simulink model "buffer_tester"  (R2024b)
settings: Solver=ode1  StartTime=0.0  StopTime=100  FixedStep=0.05  RelTol=1e-3
libraries: buffer_lib x2, filter_lib x1, storage_lib x1
settings Model: Creator=marcv  LastModifiedBy=marcv
settings RTWCC: GPUComputeCapability=3.5

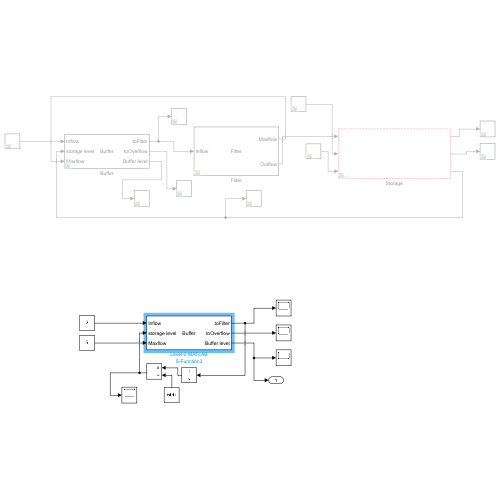
[thumbnail: Simulink's stored preview of the top-level diagram]
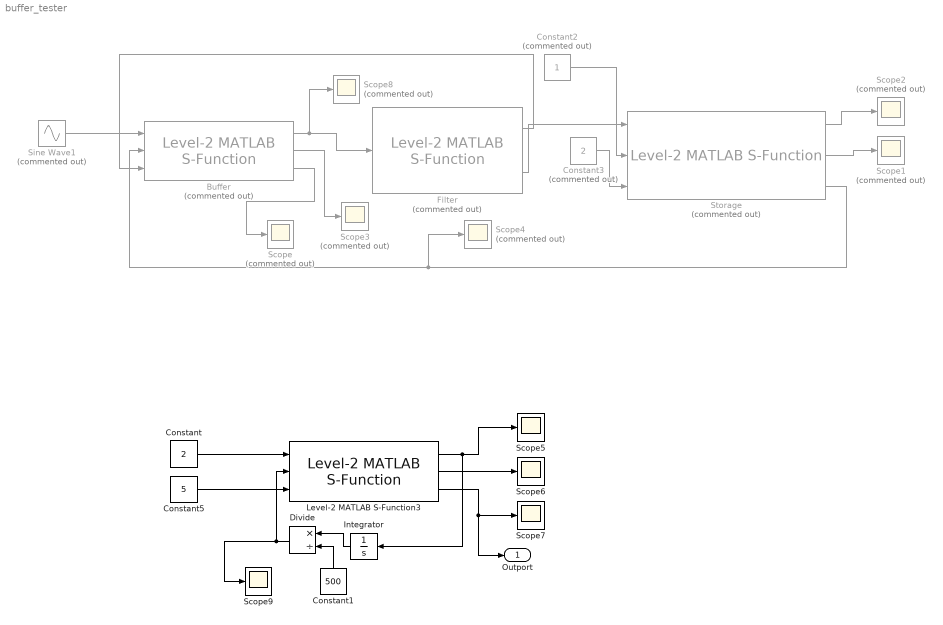
== system buffer_tester ==
  Buffer : buffer_lib/Level-2 MATLAB S-Function  Commented=on  Parameter1=100
  Constant : Constant  Value=2
  Constant1 : Constant  Value=500
  Constant2 : Constant  Commented=on
  Constant3 : Constant  Commented=on  Value=2
  Constant5 : Constant  Value=5
  Divide : Product  Inputs=*/
  Filter : filter_lib/Level-2 MATLAB S-Function  Commented=on  filteroption=Common filter  Parameter4=Cyclone-sand-UV [90 m3/h]  Parameter1=5  Parameter2=3
  Integrator : Integrator
  Level-2 MATLAB S-Function3 : buffer_lib/Level-2 MATLAB S-Function  Parameter1=1
  Scope{,1..4,8} (6 alike) : Scope  Commented=on
  Scope{5..7,9} (4 alike) : Scope
  Sine Wave1 : Sin  Commented=on  Amplitude=5  SampleTime=0
  Storage : storage_lib/Level-2 MATLAB S-Function  Commented=on  Parameter1=1000  Parameter2=0.20  Parameter3=No interconnection
  Outport : Outport
  wires:
  Sine Wave1/1 -> Buffer/1
  Buffer/2 -> Scope3/1
  Buffer/3 -> Scope/1
  Storage/3 -> Scope4/1, Buffer/2
  Storage/2 -> Scope1/1
  Constant2/1 -> Storage/2
  Constant3/1 -> Storage/3
  Storage/1 -> Scope2/1
  Buffer/1 -> Scope8/1, Filter/1
  Filter/2 -> Storage/1
  Filter/1 -> Buffer/3
  Divide/1 -> Scope9/1, Level-2 MATLAB S-Function3/2
  Constant5/1 -> Level-2 MATLAB S-Function3/3
  Constant/1 -> Level-2 MATLAB S-Function3/1
  Level-2 MATLAB S-Function3/1 -> Integrator/1, Scope5/1
  Level-2 MATLAB S-Function3/2 -> Scope6/1
  Level-2 MATLAB S-Function3/3 -> Outport/1, Scope7/1
  Integrator/1 -> Divide/1
  Constant1/1 -> Divide/2
